simulink model "diracFn2"  (R2024a)
settings: Solver=VariableStepAuto  StartTime=0.0  StopTime=10.0  RelTol=1e-3
libraries: dspsrcs4 x1
settings Model: Creator=pouya  LastModifiedBy=pouya

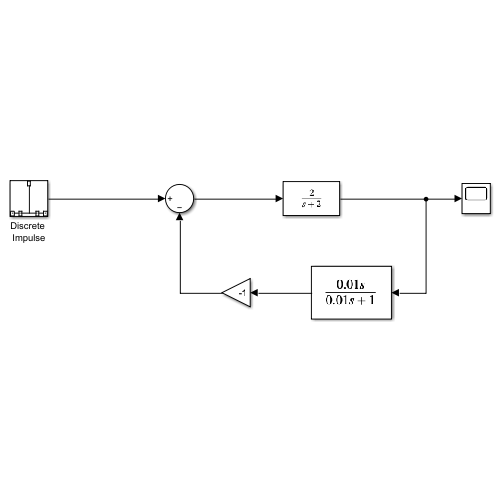
[thumbnail: Simulink's stored preview of the top-level diagram]
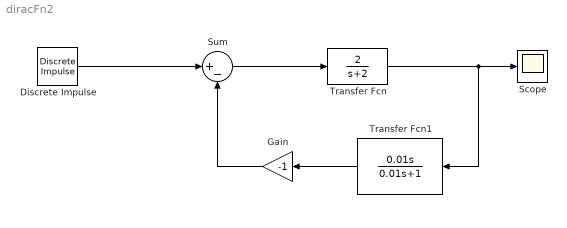
== system diracFn2 ==
  Discrete Impulse : dspsrcs4/Discrete  Impulse  Delay=0  SampleTime=1  FrameSample=1  OutputFrames=off  dataType=double  isSigned=on  wordLen=16  udDataType=sfix(16)  fracBitsMode=Best precision  numFracBits=15  OutDataTypeStr=double  LastOutDataTypeStr=double
  Gain : Gain  Gain=-1
  Scope : Scope
  Sum : Sum  Inputs=|+-
  Transfer Fcn : TransferFcn  Numerator=[2]  Denominator=[1 2]
  Transfer Fcn1 : TransferFcn  Numerator=[0.01 0]  Denominator=[0.01 1]  ParameterTunability=Unconstrained
  wires:
  Gain/1 -> Sum/2
  Transfer Fcn/1 -> Transfer Fcn1/1, Scope/1
  Sum/1 -> Transfer Fcn/1
  Transfer Fcn1/1 -> Gain/1
  Discrete Impulse/1 -> Sum/1
